simulink model "WaterPumpCtrl"  (R2018b)
settings: Solver=VariableStepAuto  StartTime=0.0  StopTime=10.0  RelTol=1e-3
libraries: simulink x5
settings Model: Creator=12045  LastModifiedBy=12045

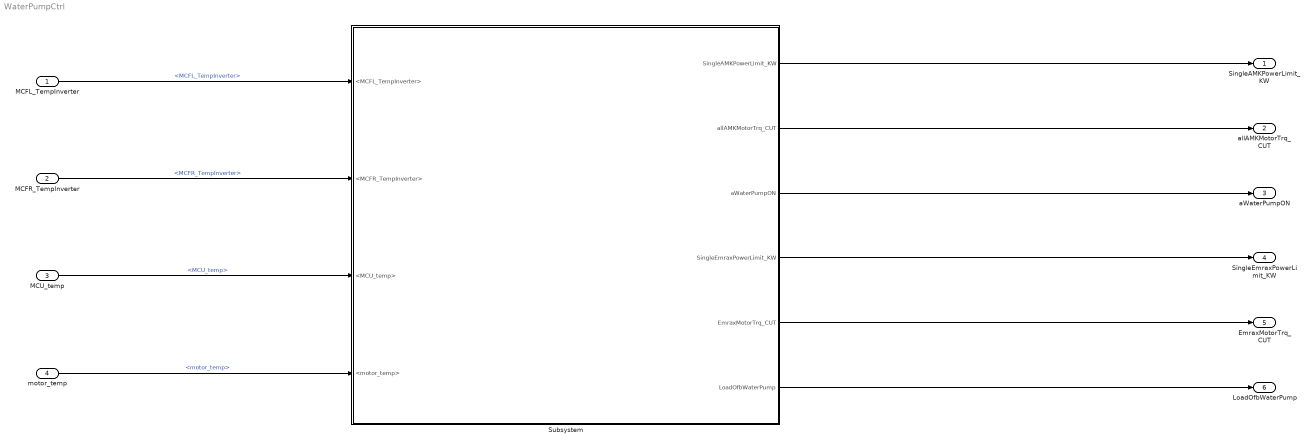
== system WaterPumpCtrl ==
  MCFL_TempInverter : Inport
  MCFR_TempInverter : Inport  Port=2
  MCU_temp : Inport  Port=3
  motor_temp : Inport  Port=4
  Subsystem : Subsystem
  SingleAMKPowerLimit_KW : Outport
  allAMKMotorTrq_CUT : Outport  Port=2
  aWaterPumpON : Outport  Port=3
  SingleEmraxPowerLimit_KW : Outport  Port=4
  EmraxMotorTrq_CUT : Outport  Port=5
  LoadOfbWaterPump : Outport  Port=6
  wires:
  MCFL_TempInverter/1 -> Subsystem/1(<MCFL_TempInverter>)  "<MCFL_TempInverter>"
  MCFR_TempInverter/1 -> Subsystem/2(<MCFR_TempInverter>)  "<MCFR_TempInverter>"
  MCU_temp/1 -> Subsystem/3(<MCU_temp>)  "<MCU_temp>"
  motor_temp/1 -> Subsystem/4(<motor_temp>)  "<motor_temp>"
  Subsystem/1(SingleAMKPowerLimit_KW) -> SingleAMKPowerLimit_KW/1
  Subsystem/2(allAMKMotorTrq_CUT) -> allAMKMotorTrq_CUT/1
  Subsystem/3(aWaterPumpON) -> aWaterPumpON/1
  Subsystem/4(SingleEmraxPowerLimit_KW) -> SingleEmraxPowerLimit_KW/1
  Subsystem/5(EmraxMotorTrq_CUT) -> EmraxMotorTrq_CUT/1
  Subsystem/6(LoadOfbWaterPump) -> LoadOfbWaterPump/1

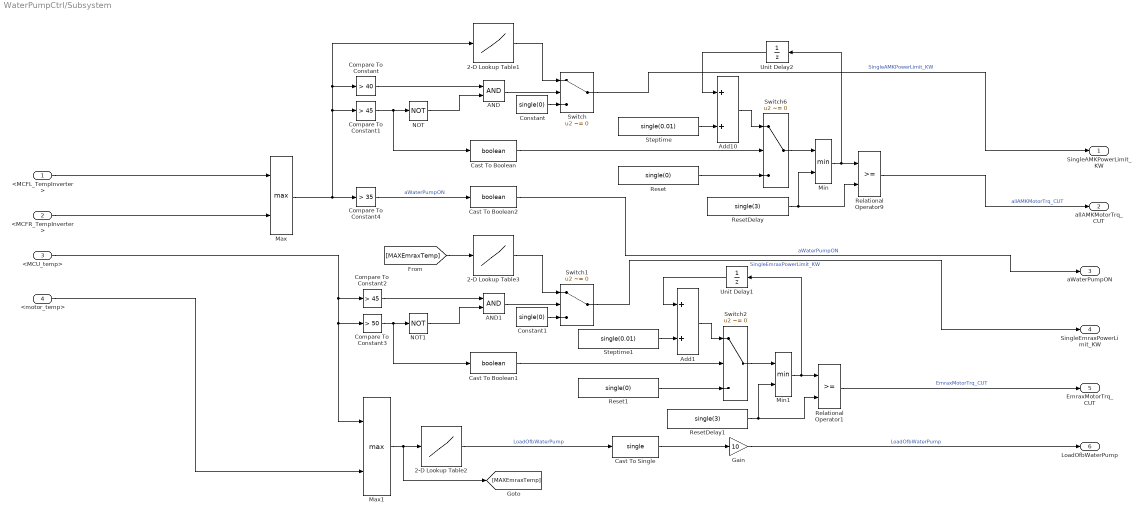
== system WaterPumpCtrl/Subsystem ==
  <MCFL_TempInverter> : Inport
  <MCFR_TempInverter> : Inport  Port=2
  <MCU_temp> : Inport  Port=3
  <motor_temp> : Inport  Port=4
  2-D Lookup Table1 : Lookup_n-D  NumberOfTableDimensions=1  BreakpointsForDimension1=[35,40,41,42,43,44,45,50]  BreakpointsForDimension2=[1:3]  Table=[0,0,0.2,0.4,0.6,0.8,1,1]  InternalRulePriority=Speed  RndMeth=Simplest  InputSameDT=on
  2-D Lookup Table2 : Lookup_n-D  NumberOfTableDimensions=1  BreakpointsForDimension1=[0;25;30;35;37;40;50]  BreakpointsForDimension2=[1:3]  Table=[0;0;20;40;70;100;100]  InternalRulePriority=Speed  RndMeth=Simplest  InputSameDT=on
  2-D Lookup Table3 : Lookup_n-D  NumberOfTableDimensions=1  BreakpointsForDimension1=[35,40,41,42,43,44,45,50]  BreakpointsForDimension2=[1:3]  Table=[0,0,0.2,0.4,0.6,0.8,1,1]  InternalRulePriority=Speed  RndMeth=Simplest  InputSameDT=on
  AND : Logic  AllPortsSameDT=off  OutDataTypeStr=boolean
  AND1 : Logic  AllPortsSameDT=off  OutDataTypeStr=boolean
  Add1 : Sum
  Add10 : Sum
  Cast To Boolean : DataTypeConversion  OutDataTypeStr=boolean
  Cast To Boolean1 : DataTypeConversion  OutDataTypeStr=boolean
  Cast To Boolean2 : DataTypeConversion  OutDataTypeStr=boolean
  Cast To Single : DataTypeConversion  OutDataTypeStr=single
  Compare To Constant : simulink/Logic and Bit Operations/Compare To Constant  relop=>  const=40  OutDataTypeStr=boolean
  Compare To Constant1 : simulink/Logic and Bit Operations/Compare To Constant  relop=>  const=45  OutDataTypeStr=boolean
  Compare To Constant2 : simulink/Logic and Bit Operations/Compare To Constant  relop=>  const=45  OutDataTypeStr=boolean
  Compare To Constant3 : simulink/Logic and Bit Operations/Compare To Constant  relop=>  const=50  OutDataTypeStr=boolean
  Compare To Constant4 : simulink/Logic and Bit Operations/Compare To Constant  relop=>  const=35  OutDataTypeStr=boolean
  Constant : Constant  Value=single(0)
  Constant1 : Constant  Value=single(0)
  Gain : Gain  Gain=10
  Max : MinMax  Function=max  Inputs=2
  Max1 : MinMax  Function=max  Inputs=2
  Min : MinMax  Inputs=2
  Min1 : MinMax  Inputs=2
  NOT : Logic  Operator=NOT  AllPortsSameDT=off  OutDataTypeStr=boolean
  NOT1 : Logic  Operator=NOT  AllPortsSameDT=off  OutDataTypeStr=boolean
  Relational Operator1 : RelationalOperator  OutDataTypeStr=boolean  RndMeth=Simplest
  Relational Operator9 : RelationalOperator  OutDataTypeStr=boolean  RndMeth=Simplest
  Reset : Constant  Value=single(0)
  Reset1 : Constant  Value=single(0)
  ResetDelay : Constant  Value=single(3)
  ResetDelay1 : Constant  Value=single(3)
  Steptime : Constant  Value=single(0.01)
  Steptime1 : Constant  Value=single(0.01)
  Switch{,1..2,6} (4 alike) : Switch  Criteria=u2 ~= 0
  Unit Delay1 : UnitDelay  SampleTime=-1
  Unit Delay2 : UnitDelay  SampleTime=-1
  SingleAMKPowerLimit_KW : Outport
  allAMKMotorTrq_CUT : Outport  Port=2
  aWaterPumpON : Outport  Port=3
  SingleEmraxPowerLimit_KW : Outport  Port=4
  EmraxMotorTrq_CUT : Outport  Port=5
  LoadOfbWaterPump : Outport  Port=6
  wires:
  Min1/1 -> Unit Delay1/1, Relational Operator1/1
  Unit Delay1/1 -> Add1/1
  Relational Operator9/1 -> allAMKMotorTrq_CUT/1  "allAMKMotorTrq_CUT"
  Switch2/1 -> Min1/1
  Min/1 -> Relational Operator9/1, Unit Delay2/1
  Switch6/1 -> Min/1
  Steptime/1 -> Add10/2
  <MCU_temp>/1 -> Max1/1, Compare To Constant3/1, Compare To Constant2/1
  Reset/1 -> Switch6/3
  AND1/1 -> Switch1/2
  Compare To Constant2/1 -> AND1/1
  2-D Lookup Table2/1 -> Cast To Single/1  "LoadOfbWaterPump"
  Add1/1 -> Switch2/1
  Max/1 -> Compare To Constant4/1, 2-D Lookup Table1/1, Compare To Constant/1, Compare To Constant1/1
  AND/1 -> Switch/2
  NOT/1 -> AND/2
  Compare To Constant3/1 -> NOT1/1, Cast To Boolean1/1
  Cast To Single/1 -> Gain/1
  Constant/1 -> Switch/3
  Max1/1 -> [MAXEmraxTemp], 2-D Lookup Table2/1
  Compare To Constant1/1 -> Cast To Boolean/1, NOT/1
  NOT1/1 -> AND1/2
  2-D Lookup Table3/1 -> Switch1/1
  Reset1/1 -> Switch2/3
  Cast To Boolean/1 -> Switch6/2
  Steptime1/1 -> Add1/2
  ResetDelay1/1 -> Min1/2, Relational Operator1/2
  Unit Delay2/1 -> Add10/1
  ResetDelay/1 -> Relational Operator9/2, Min/2
  Switch1/1 -> SingleEmraxPowerLimit_KW/1  "SingleEmraxPowerLimit_KW"
  <motor_temp>/1 -> Max1/2
  Constant1/1 -> Switch1/3
  Cast To Boolean1/1 -> Switch2/2
  <MCFL_TempInverter>/1 -> Max/1
  <MCFR_TempInverter>/1 -> Max/2
  Compare To Constant/1 -> AND/1
  Compare To Constant4/1 -> Cast To Boolean2/1  "aWaterPumpON"
  [MAXEmraxTemp] -> 2-D Lookup Table3/1
  2-D Lookup Table1/1 -> Switch/1
  Cast To Boolean2/1 -> aWaterPumpON/1  "aWaterPumpON"
  Add10/1 -> Switch6/1
  Gain/1 -> LoadOfbWaterPump/1  "LoadOfbWaterPump"
  Relational Operator1/1 -> EmraxMotorTrq_CUT/1  "EmraxMotorTrq_CUT"
  Switch/1 -> SingleAMKPowerLimit_KW/1  "SingleAMKPowerLimit_KW"
